simulink model "component_model"  (R2019a)
settings: Solver=VariableStepAuto  StartTime=0.0  StopTime=10.0  RelTol=1e-3
settings Model: Creator=anton  LastModifiedBy=anton

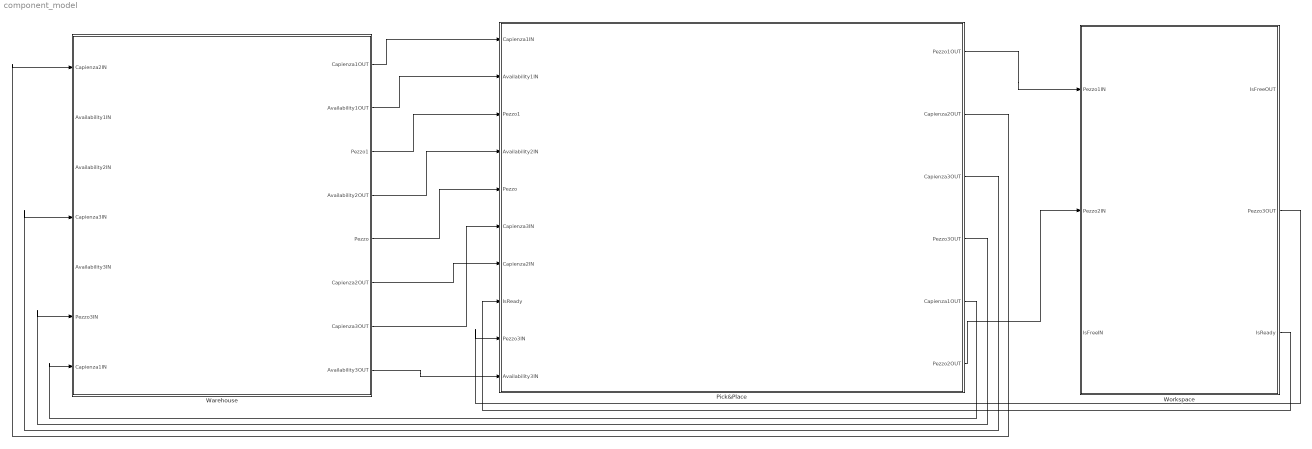
== system component_model ==
  Pick&Place : Subsystem
      settings: PortSchema="{\"entries\":[{\"content\":{\"headerSize\":26,\"margin\":15,\"minimumSpacing\":25,\"sides\":[{\"content\":{\"connectorIds\":[\"In1\",\"In2\",\"In3\",\"In4\",\"In5\",\"In6\",\"In7\",\"In8\",\"In9\",\"In10\"]},\"type\":\"ConnectorPlacement.EquallySpacedRectSide\",\"uuid\":\"cd5611c0-8a30-4803-bae5-8792d5ed3138\"},{\"content\":{\"connectorIds\":[\"Out1\",\"Out2\",\"Out3\",\"Out4\",\"Out5\",\"Out6\"],\"side\":\"RIGHT\"},\"type\":\"ConnectorPlacement.EquallySpacedRectSide\",\"uuid\":\"19615e04-708c-4dc8-9217-130af3d4c815\"},{\"content\":{\"connectorIds\":[],\"side\":\"TOP\"},\"type\":\"ConnectorPlacement.EquallySpacedRectSide\",\"uuid\":\"bde4fae3-4c2b-4ff8-8efa-5dc73cdd4226\"}]},\"type\":\"ConnectorPlacement.EquallySpacedConnector\",\"uuid\":\"74f0ebde-c382-4fb1-af99-ecf6372bc12c\"}],\"packageUris\":[\"http:\\/\\/schema.mathworks.com\\/mf0\\/Connector\\/19700101\"],\"version\":\"1.0\"}"
  Warehouse : Subsystem
      settings: PortSchema="{\"entries\":[{\"content\":{\"headerSize\":26,\"margin\":15,\"minimumSpacing\":25,\"sides\":[{\"content\":{\"connectorIds\":[\"In1\",\"In2\",\"In3\",\"In4\",\"In5\",\"In6\",\"In7\"]},\"type\":\"ConnectorPlacement.EquallySpacedRectSide\",\"uuid\":\"cd5611c0-8a30-4803-bae5-8792d5ed3138\"},{\"content\":{\"connectorIds\":[\"Out1\",\"Out2\",\"Out3\",\"Out4\",\"Out5\",\"Out6\",\"Out7\",\"Out8\"],\"side\":\"RIGHT\"},\"type\":\"ConnectorPlacement.EquallySpacedRectSide\",\"uuid\":\"19615e04-708c-4dc8-9217-130af3d4c815\"},{\"content\":{\"connectorIds\":[],\"side\":\"TOP\"},\"type\":\"ConnectorPlacement.EquallySpacedRectSide\",\"uuid\":\"bde4fae3-4c2b-4ff8-8efa-5dc73cdd4226\"}]},\"type\":\"ConnectorPlacement.EquallySpacedConnector\",\"uuid\":\"74f0ebde-c382-4fb1-af99-ecf6372bc12c\"}],\"packageUris\":[\"http:\\/\\/schema.mathworks.com\\/mf0\\/Connector\\/19700101\"],\"version\":\"1.0\"}"
  Workspace : Subsystem
      settings: PortSchema="{\"entries\":[{\"content\":{\"headerSize\":26,\"margin\":15,\"minimumSpacing\":25,\"sides\":[{\"content\":{\"connectorIds\":[\"In1\",\"In2\",\"In3\"]},\"type\":\"ConnectorPlacement.EquallySpacedRectSide\",\"uuid\":\"cd5611c0-8a30-4803-bae5-8792d5ed3138\"},{\"content\":{\"connectorIds\":[\"Out1\",\"Out2\",\"Out3\"],\"side\":\"RIGHT\"},\"type\":\"ConnectorPlacement.EquallySpacedRectSide\",\"uuid\":\"19615e04-708c-4dc8-9217-130af3d4c815\"},{\"content\":{\"connectorIds\":[],\"side\":\"TOP\"},\"type\":\"ConnectorPlacement.EquallySpacedRectSide\",\"uuid\":\"bde4fae3-4c2b-4ff8-8efa-5dc73cdd4226\"}]},\"type\":\"ConnectorPlacement.EquallySpacedConnector\",\"uuid\":\"74f0ebde-c382-4fb1-af99-ecf6372bc12c\"}],\"packageUris\":[\"http:\\/\\/schema.mathworks.com\\/mf0\\/Connector\\/19700101\"],\"version\":\"1.0\"}"
  wires:
  Pick&Place/5(Capienza1OUT) -> Warehouse/7(Capienza1IN)
  Pick&Place/2(Capienza2OUT) -> Warehouse/1(Capienza2IN)
  Pick&Place/3(Capienza3OUT) -> Warehouse/4(Capienza3IN)
  Warehouse/1(Capienza1OUT) -> Pick&Place/1(Capienza1IN)
  Warehouse/6(Capienza2OUT) -> Pick&Place/7(Capienza2IN)
  Warehouse/3(Pezzo1) -> Pick&Place/3(Pezzo1)
  Warehouse/5(Pezzo) -> Pick&Place/5(Pezzo)
  Warehouse/2(Availability1OUT) -> Pick&Place/2(Availability1IN)
  Warehouse/4(Availability2OUT) -> Pick&Place/4(Availability2IN)
  Warehouse/7(Capienza3OUT) -> Pick&Place/6(Capienza3IN)
  Pick&Place/1(Pezzo1OUT) -> Workspace/1(Pezzo1IN)
  Pick&Place/6(Pezzo2OUT) -> Workspace/2(Pezzo2IN)
  Workspace/3(IsReady) -> Pick&Place/8(IsReady)
  Workspace/2(Pezzo3OUT) -> Pick&Place/9(Pezzo3IN)
  Pick&Place/4(Pezzo3OUT) -> Warehouse/6(Pezzo3IN)
  Warehouse/8(Availability3OUT) -> Pick&Place/10(Availability3IN)

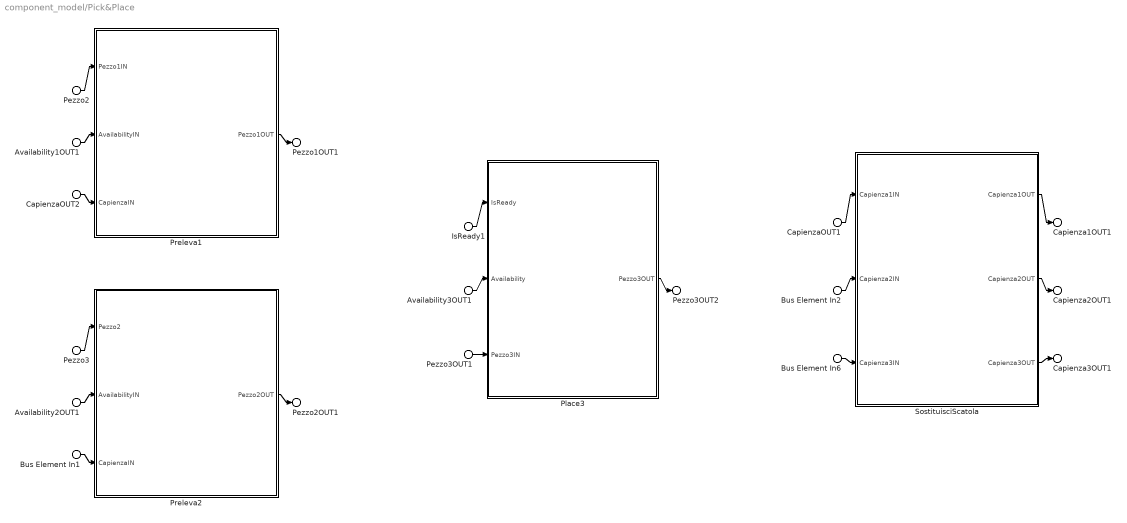
== system component_model/Pick&Place ==
  CapienzaOUT1 : Inport  PortName=Capienza1IN
  CapienzaOUT2 : Inport  PortName=Capienza1IN
  Availability1OUT1 : Inport  Port=2  PortName=Availability1IN
  Pezzo2 : Inport  Port=3  PortName=Pezzo1
  Availability2OUT1 : Inport  Port=4  PortName=Availability2IN
  Pezzo3 : Inport  Port=5  PortName=Pezzo
  Bus Element In6 : Inport  Port=6  PortName=Capienza3IN
  Bus Element In2 : Inport  Port=7  PortName=Capienza2IN
  Bus Element In1 : Inport  Port=7  PortName=Capienza2IN
  IsReady1 : Inport  Port=8  PortName=IsReady
  Pezzo3OUT1 : Inport  Port=9  PortName=Pezzo3IN
  Availability3OUT1 : Inport  Port=10  PortName=Availability3IN
  Place3 : Subsystem
      settings: PortSchema="{\"entries\":[{\"content\":{\"headerSize\":26,\"margin\":15,\"minimumSpacing\":25,\"sides\":[{\"content\":{\"connectorIds\":[\"In1\",\"In2\",\"In3\"]},\"type\":\"ConnectorPlacement.EquallySpacedRectSide\",\"uuid\":\"cd5611c0-8a30-4803-bae5-8792d5ed3138\"},{\"content\":{\"connectorIds\":[\"Out1\"],\"side\":\"RIGHT\"},\"type\":\"ConnectorPlacement.EquallySpacedRectSide\",\"uuid\":\"19615e04-708c-4dc8-9217-130af3d4c815\"},{\"content\":{\"connectorIds\":[],\"side\":\"TOP\"},\"type\":\"ConnectorPlacement.EquallySpacedRectSide\",\"uuid\":\"bde4fae3-4c2b-4ff8-8efa-5dc73cdd4226\"},{\"content\":{\"connectorIds\":[],\"side\":\"BOTTOM\"},\"type\":\"ConnectorPlacement.EquallySpacedRectSide\",\"uuid\":\"1c0666f0-126c-43a7-b404-605aac664503\"}]},\"type\":\"ConnectorPlacement.EquallySpacedConnector\",\"uuid\":\"74f0ebde-c382-4fb1-af99-ecf6372bc12c\"}],\"packageUris\":[\"http:\\/\\/schema.mathworks.com\\/mf0\\/Connector\\/19700101\"],\"version\":\"1.0\"}"
  Preleva1 : Subsystem
      settings: PortSchema="{\"entries\":[{\"content\":{\"headerSize\":26,\"margin\":15,\"minimumSpacing\":25,\"sides\":[{\"content\":{\"connectorIds\":[\"In1\",\"In2\",\"In3\"]},\"type\":\"ConnectorPlacement.EquallySpacedRectSide\",\"uuid\":\"cd5611c0-8a30-4803-bae5-8792d5ed3138\"},{\"content\":{\"connectorIds\":[\"Out1\"],\"side\":\"RIGHT\"},\"type\":\"ConnectorPlacement.EquallySpacedRectSide\",\"uuid\":\"19615e04-708c-4dc8-9217-130af3d4c815\"},{\"content\":{\"connectorIds\":[],\"side\":\"TOP\"},\"type\":\"ConnectorPlacement.EquallySpacedRectSide\",\"uuid\":\"bde4fae3-4c2b-4ff8-8efa-5dc73cdd4226\"}]},\"type\":\"ConnectorPlacement.EquallySpacedConnector\",\"uuid\":\"74f0ebde-c382-4fb1-af99-ecf6372bc12c\"}],\"packageUris\":[\"http:\\/\\/schema.mathworks.com\\/mf0\\/Connector\\/19700101\"],\"version\":\"1.0\"}"
  Preleva2 : Subsystem
      settings: PortSchema="{\"entries\":[{\"content\":{\"headerSize\":26,\"margin\":15,\"minimumSpacing\":25,\"sides\":[{\"content\":{\"connectorIds\":[\"In1\",\"In2\",\"In3\"]},\"type\":\"ConnectorPlacement.EquallySpacedRectSide\",\"uuid\":\"cd5611c0-8a30-4803-bae5-8792d5ed3138\"},{\"content\":{\"connectorIds\":[\"Out1\"],\"side\":\"RIGHT\"},\"type\":\"ConnectorPlacement.EquallySpacedRectSide\",\"uuid\":\"19615e04-708c-4dc8-9217-130af3d4c815\"},{\"content\":{\"connectorIds\":[],\"side\":\"TOP\"},\"type\":\"ConnectorPlacement.EquallySpacedRectSide\",\"uuid\":\"bde4fae3-4c2b-4ff8-8efa-5dc73cdd4226\"}]},\"type\":\"ConnectorPlacement.EquallySpacedConnector\",\"uuid\":\"74f0ebde-c382-4fb1-af99-ecf6372bc12c\"}],\"packageUris\":[\"http:\\/\\/schema.mathworks.com\\/mf0\\/Connector\\/19700101\"],\"version\":\"1.0\"}"
  SostituisciScatola : Subsystem
      settings: PortSchema="{\"entries\":[{\"content\":{\"headerSize\":26,\"margin\":15,\"minimumSpacing\":25,\"sides\":[{\"content\":{\"connectorIds\":[\"In1\",\"In2\",\"In3\"]},\"type\":\"ConnectorPlacement.EquallySpacedRectSide\",\"uuid\":\"cd5611c0-8a30-4803-bae5-8792d5ed3138\"},{\"content\":{\"connectorIds\":[\"Out1\",\"Out2\",\"Out3\"],\"side\":\"RIGHT\"},\"type\":\"ConnectorPlacement.EquallySpacedRectSide\",\"uuid\":\"19615e04-708c-4dc8-9217-130af3d4c815\"},{\"content\":{\"connectorIds\":[],\"side\":\"TOP\"},\"type\":\"ConnectorPlacement.EquallySpacedRectSide\",\"uuid\":\"bde4fae3-4c2b-4ff8-8efa-5dc73cdd4226\"}]},\"type\":\"ConnectorPlacement.EquallySpacedConnector\",\"uuid\":\"74f0ebde-c382-4fb1-af99-ecf6372bc12c\"}],\"packageUris\":[\"http:\\/\\/schema.mathworks.com\\/mf0\\/Connector\\/19700101\"],\"version\":\"1.0\"}"
  Pezzo1OUT1 : Outport  PortName=Pezzo1OUT
  Capienza2OUT1 : Outport  Port=2  PortName=Capienza2OUT
  Capienza3OUT1 : Outport  Port=3  PortName=Capienza3OUT
  Pezzo3OUT2 : Outport  Port=4  PortName=Pezzo3OUT
  Capienza1OUT1 : Outport  Port=5  PortName=Capienza1OUT
  Pezzo2OUT1 : Outport  Port=6  PortName=Pezzo2OUT
  wires:
  SostituisciScatola/1(Capienza1OUT) -> Capienza1OUT1/1
  SostituisciScatola/2(Capienza2OUT) -> Capienza2OUT1/1
  SostituisciScatola/3(Capienza3OUT) -> Capienza3OUT1/1
  CapienzaOUT1/1 -> SostituisciScatola/1(Capienza1IN)
  Bus Element In2/1 -> SostituisciScatola/2(Capienza2IN)
  CapienzaOUT2/1 -> Preleva1/3(CapienzaIN)
  Bus Element In1/1 -> Preleva2/3(CapienzaIN)
  Pezzo2/1 -> Preleva1/1(Pezzo1IN)
  Pezzo3/1 -> Preleva2/1(Pezzo2)
  Availability1OUT1/1 -> Preleva1/2(AvailabilityIN)
  Availability2OUT1/1 -> Preleva2/2(AvailabilityIN)
  Preleva1/1(Pezzo1OUT) -> Pezzo1OUT1/1
  Preleva2/1(Pezzo2OUT) -> Pezzo2OUT1/1
  Bus Element In6/1 -> SostituisciScatola/3(Capienza3IN)
  IsReady1/1 -> Place3/1(IsReady)
  Pezzo3OUT1/1 -> Place3/3(Pezzo3IN)
  Place3/1(Pezzo3OUT) -> Pezzo3OUT2/1
  Availability3OUT1/1 -> Place3/2(Availability)

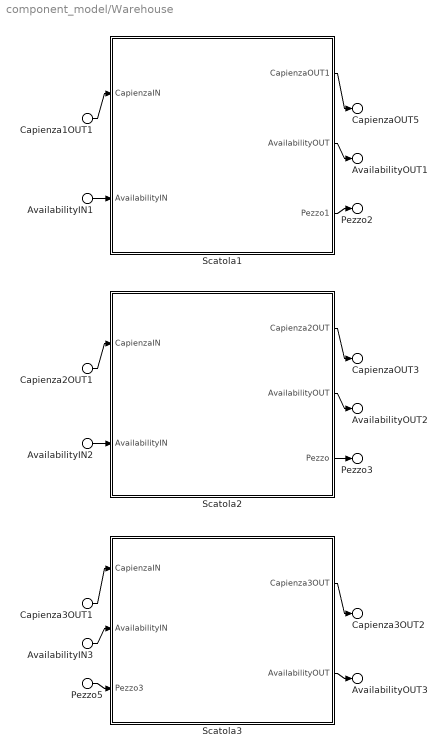
== system component_model/Warehouse ==
  Capienza2OUT1 : Inport  PortName=Capienza2IN
  AvailabilityIN1 : Inport  Port=2  PortName=Availability1IN
  AvailabilityIN2 : Inport  Port=3  PortName=Availability2IN
  Capienza3OUT1 : Inport  Port=4  PortName=Capienza3IN
  AvailabilityIN3 : Inport  Port=5  PortName=Availability3IN
  Pezzo5 : Inport  Port=6  PortName=Pezzo3IN
  Capienza1OUT1 : Inport  Port=7  PortName=Capienza1IN
  Scatola1 : Subsystem
      settings: PortSchema="{\"entries\":[{\"content\":{\"headerSize\":26,\"margin\":15,\"minimumSpacing\":25,\"sides\":[{\"content\":{\"connectorIds\":[\"In1\",\"In2\"]},\"type\":\"ConnectorPlacement.EquallySpacedRectSide\",\"uuid\":\"cd5611c0-8a30-4803-bae5-8792d5ed3138\"},{\"content\":{\"connectorIds\":[\"Out1\",\"Out2\",\"Out3\"],\"side\":\"RIGHT\"},\"type\":\"ConnectorPlacement.EquallySpacedRectSide\",\"uuid\":\"19615e04-708c-4dc8-9217-130af3d4c815\"},{\"content\":{\"connectorIds\":[],\"side\":\"TOP\"},\"type\":\"ConnectorPlacement.EquallySpacedRectSide\",\"uuid\":\"bde4fae3-4c2b-4ff8-8efa-5dc73cdd4226\"}]},\"type\":\"ConnectorPlacement.EquallySpacedConnector\",\"uuid\":\"74f0ebde-c382-4fb1-af99-ecf6372bc12c\"}],\"packageUris\":[\"http:\\/\\/schema.mathworks.com\\/mf0\\/Connector\\/19700101\"],\"version\":\"1.0\"}"
  Scatola2 : Subsystem
      settings: PortSchema="{\"entries\":[{\"content\":{\"headerSize\":26,\"margin\":15,\"minimumSpacing\":25,\"sides\":[{\"content\":{\"connectorIds\":[\"In1\",\"In2\"]},\"type\":\"ConnectorPlacement.EquallySpacedRectSide\",\"uuid\":\"cd5611c0-8a30-4803-bae5-8792d5ed3138\"},{\"content\":{\"connectorIds\":[\"Out1\",\"Out2\",\"Out3\"],\"side\":\"RIGHT\"},\"type\":\"ConnectorPlacement.EquallySpacedRectSide\",\"uuid\":\"19615e04-708c-4dc8-9217-130af3d4c815\"},{\"content\":{\"connectorIds\":[],\"side\":\"TOP\"},\"type\":\"ConnectorPlacement.EquallySpacedRectSide\",\"uuid\":\"bde4fae3-4c2b-4ff8-8efa-5dc73cdd4226\"}]},\"type\":\"ConnectorPlacement.EquallySpacedConnector\",\"uuid\":\"74f0ebde-c382-4fb1-af99-ecf6372bc12c\"}],\"packageUris\":[\"http:\\/\\/schema.mathworks.com\\/mf0\\/Connector\\/19700101\"],\"version\":\"1.0\"}"
  Scatola3 : Subsystem
      settings: PortSchema="{\"entries\":[{\"content\":{\"headerSize\":26,\"margin\":15,\"minimumSpacing\":25,\"sides\":[{\"content\":{\"connectorIds\":[\"In1\",\"In2\",\"In3\"]},\"type\":\"ConnectorPlacement.EquallySpacedRectSide\",\"uuid\":\"cd5611c0-8a30-4803-bae5-8792d5ed3138\"},{\"content\":{\"connectorIds\":[\"Out1\",\"Out2\"],\"side\":\"RIGHT\"},\"type\":\"ConnectorPlacement.EquallySpacedRectSide\",\"uuid\":\"19615e04-708c-4dc8-9217-130af3d4c815\"},{\"content\":{\"connectorIds\":[],\"side\":\"TOP\"},\"type\":\"ConnectorPlacement.EquallySpacedRectSide\",\"uuid\":\"bde4fae3-4c2b-4ff8-8efa-5dc73cdd4226\"}]},\"type\":\"ConnectorPlacement.EquallySpacedConnector\",\"uuid\":\"74f0ebde-c382-4fb1-af99-ecf6372bc12c\"}],\"packageUris\":[\"http:\\/\\/schema.mathworks.com\\/mf0\\/Connector\\/19700101\"],\"version\":\"1.0\"}"
  CapienzaOUT5 : Outport  PortName=Capienza1OUT
  AvailabilityOUT1 : Outport  Port=2  PortName=Availability1OUT
  Pezzo2 : Outport  Port=3  PortName=Pezzo1
  AvailabilityOUT2 : Outport  Port=4  PortName=Availability2OUT
  Pezzo3 : Outport  Port=5  PortName=Pezzo
  CapienzaOUT3 : Outport  Port=6  PortName=Capienza2OUT
  Capienza3OUT2 : Outport  Port=7  PortName=Capienza3OUT
  AvailabilityOUT3 : Outport  Port=8  PortName=Availability3OUT
  wires:
  Capienza3OUT1/1 -> Scatola3/1(CapienzaIN)
  Capienza1OUT1/1 -> Scatola1/1(CapienzaIN)
  Capienza2OUT1/1 -> Scatola2/1(CapienzaIN)
  Scatola2/1(Capienza2OUT) -> CapienzaOUT3/1
  Scatola1/1(CapienzaOUT1) -> CapienzaOUT5/1
  Scatola1/2(AvailabilityOUT) -> AvailabilityOUT1/1
  Scatola2/2(AvailabilityOUT) -> AvailabilityOUT2/1
  Scatola3/2(AvailabilityOUT) -> AvailabilityOUT3/1
  Scatola1/3(Pezzo1) -> Pezzo2/1
  Scatola2/3(Pezzo) -> Pezzo3/1
  Scatola3/1(Capienza3OUT) -> Capienza3OUT2/1
  AvailabilityIN1/1 -> Scatola1/2(AvailabilityIN)
  AvailabilityIN2/1 -> Scatola2/2(AvailabilityIN)
  AvailabilityIN3/1 -> Scatola3/2(AvailabilityIN)
  Pezzo5/1 -> Scatola3/3(Pezzo3)

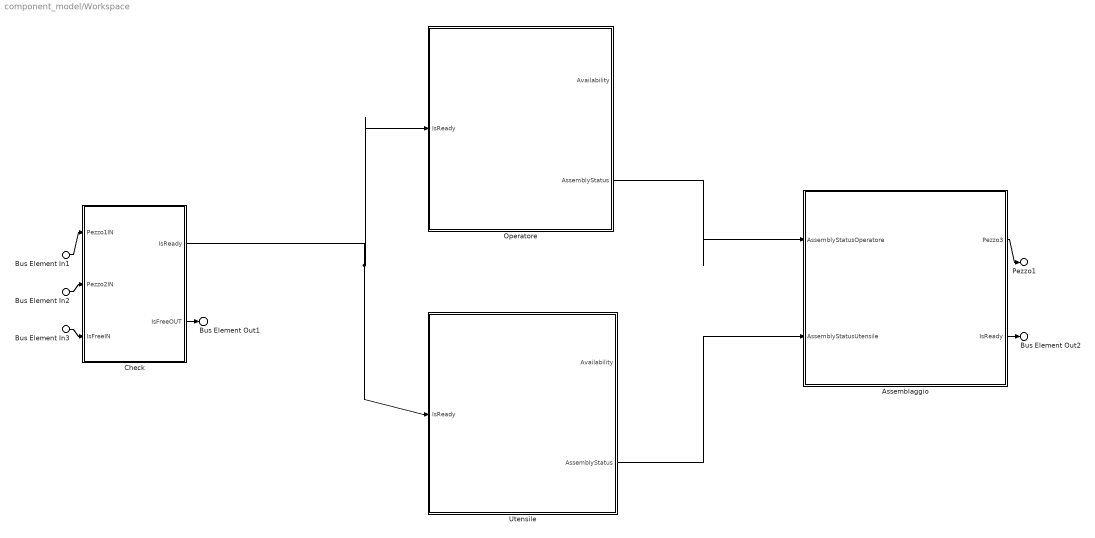
== system component_model/Workspace ==
  Bus Element In1 : Inport  PortName=Pezzo1IN
  Bus Element In2 : Inport  Port=2  PortName=Pezzo2IN
  Bus Element In3 : Inport  Port=3  PortName=IsFreeIN
  Assemblaggio : Subsystem
      settings: PortSchema="{\"entries\":[{\"content\":{\"headerSize\":26,\"margin\":15,\"minimumSpacing\":25,\"sides\":[{\"content\":{\"connectorIds\":[\"In1\",\"In2\"]},\"type\":\"ConnectorPlacement.EquallySpacedRectSide\",\"uuid\":\"cd5611c0-8a30-4803-bae5-8792d5ed3138\"},{\"content\":{\"connectorIds\":[\"Out1\",\"Out2\"],\"side\":\"RIGHT\"},\"type\":\"ConnectorPlacement.EquallySpacedRectSide\",\"uuid\":\"19615e04-708c-4dc8-9217-130af3d4c815\"},{\"content\":{\"connectorIds\":[],\"side\":\"TOP\"},\"type\":\"ConnectorPlacement.EquallySpacedRectSide\",\"uuid\":\"bde4fae3-4c2b-4ff8-8efa-5dc73cdd4226\"}]},\"type\":\"ConnectorPlacement.EquallySpacedConnector\",\"uuid\":\"74f0ebde-c382-4fb1-af99-ecf6372bc12c\"}],\"packageUris\":[\"http:\\/\\/schema.mathworks.com\\/mf0\\/Connector\\/19700101\"],\"version\":\"1.0\"}"
  Check : Subsystem
      settings: PortSchema="{\"entries\":[{\"content\":{\"headerSize\":26,\"margin\":15,\"minimumSpacing\":25,\"sides\":[{\"content\":{\"connectorIds\":[\"In1\",\"In2\",\"In3\"]},\"type\":\"ConnectorPlacement.EquallySpacedRectSide\",\"uuid\":\"cd5611c0-8a30-4803-bae5-8792d5ed3138\"},{\"content\":{\"connectorIds\":[\"Out1\",\"Out2\"],\"side\":\"RIGHT\"},\"type\":\"ConnectorPlacement.EquallySpacedRectSide\",\"uuid\":\"19615e04-708c-4dc8-9217-130af3d4c815\"},{\"content\":{\"connectorIds\":[],\"side\":\"TOP\"},\"type\":\"ConnectorPlacement.EquallySpacedRectSide\",\"uuid\":\"bde4fae3-4c2b-4ff8-8efa-5dc73cdd4226\"}]},\"type\":\"ConnectorPlacement.EquallySpacedConnector\",\"uuid\":\"74f0ebde-c382-4fb1-af99-ecf6372bc12c\"}],\"packageUris\":[\"http:\\/\\/schema.mathworks.com\\/mf0\\/Connector\\/19700101\"],\"version\":\"1.0\"}"
  Operatore : Subsystem
      settings: PortSchema="{\"entries\":[{\"content\":{\"headerSize\":26,\"margin\":15,\"minimumSpacing\":25,\"sides\":[{\"content\":{\"connectorIds\":[\"In1\"]},\"type\":\"ConnectorPlacement.EquallySpacedRectSide\",\"uuid\":\"cd5611c0-8a30-4803-bae5-8792d5ed3138\"},{\"content\":{\"connectorIds\":[\"Out1\",\"Out2\"],\"side\":\"RIGHT\"},\"type\":\"ConnectorPlacement.EquallySpacedRectSide\",\"uuid\":\"19615e04-708c-4dc8-9217-130af3d4c815\"},{\"content\":{\"connectorIds\":[],\"side\":\"TOP\"},\"type\":\"ConnectorPlacement.EquallySpacedRectSide\",\"uuid\":\"bde4fae3-4c2b-4ff8-8efa-5dc73cdd4226\"}]},\"type\":\"ConnectorPlacement.EquallySpacedConnector\",\"uuid\":\"74f0ebde-c382-4fb1-af99-ecf6372bc12c\"}],\"packageUris\":[\"http:\\/\\/schema.mathworks.com\\/mf0\\/Connector\\/19700101\"],\"version\":\"1.0\"}"
  Utensile : Subsystem
      settings: PortSchema="{\"entries\":[{\"content\":{\"headerSize\":26,\"margin\":15,\"minimumSpacing\":25,\"sides\":[{\"content\":{\"connectorIds\":[\"In1\"]},\"type\":\"ConnectorPlacement.EquallySpacedRectSide\",\"uuid\":\"cd5611c0-8a30-4803-bae5-8792d5ed3138\"},{\"content\":{\"connectorIds\":[\"Out1\",\"Out2\"],\"side\":\"RIGHT\"},\"type\":\"ConnectorPlacement.EquallySpacedRectSide\",\"uuid\":\"19615e04-708c-4dc8-9217-130af3d4c815\"},{\"content\":{\"connectorIds\":[],\"side\":\"TOP\"},\"type\":\"ConnectorPlacement.EquallySpacedRectSide\",\"uuid\":\"bde4fae3-4c2b-4ff8-8efa-5dc73cdd4226\"}]},\"type\":\"ConnectorPlacement.EquallySpacedConnector\",\"uuid\":\"74f0ebde-c382-4fb1-af99-ecf6372bc12c\"}],\"packageUris\":[\"http:\\/\\/schema.mathworks.com\\/mf0\\/Connector\\/19700101\"],\"version\":\"1.0\"}"
  Bus Element Out1 : Outport  PortName=IsFreeOUT
  Pezzo1 : Outport  Port=2  PortName=Pezzo3OUT
  Bus Element Out2 : Outport  Port=3  PortName=IsReady
  wires:
  Operatore/2(AssemblyStatus) -> Assemblaggio/1(AssemblyStatusOperatore)
  Utensile/2(AssemblyStatus) -> Assemblaggio/2(AssemblyStatusUtensile)
  Bus Element In1/1 -> Check/1(Pezzo1IN)
  Bus Element In2/1 -> Check/2(Pezzo2IN)
  Check/1(IsReady) -> Utensile/1(IsReady), Operatore/1(IsReady)
  Assemblaggio/1(Pezzo3) -> Pezzo1/1
  Assemblaggio/2(IsReady) -> Bus Element Out2/1
  Bus Element In3/1 -> Check/3(IsFreeIN)
  Check/2(IsFreeOUT) -> Bus Element Out1/1

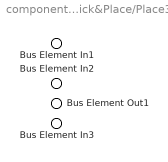
== system component_model/Pick&Place/Place3 ==
  Bus Element In1 : Inport  PortName=IsReady
  Bus Element In2 : Inport  Port=2  PortName=Availability
  Bus Element In3 : Inport  Port=3  PortName=Pezzo3IN
  Bus Element Out1 : Outport  PortName=Pezzo3OUT

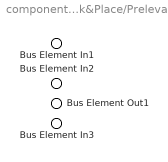
== system component_model/Pick&Place/Preleva1 ==
  Bus Element In1 : Inport  PortName=Pezzo1IN
  Bus Element In2 : Inport  Port=2  PortName=AvailabilityIN
  Bus Element In3 : Inport  Port=3  PortName=CapienzaIN
  Bus Element Out1 : Outport  PortName=Pezzo1OUT

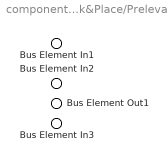
== system component_model/Pick&Place/Preleva2 ==
  Bus Element In1 : Inport  PortName=Pezzo2
  Bus Element In2 : Inport  Port=2  PortName=AvailabilityIN
  Bus Element In3 : Inport  Port=3  PortName=CapienzaIN
  Bus Element Out1 : Outport  PortName=Pezzo2OUT

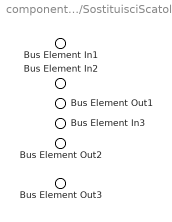
== system component_model/Pick&Place/SostituisciScatola ==
  Bus Element In1 : Inport  PortName=Capienza1IN
  Bus Element In2 : Inport  Port=2  PortName=Capienza2IN
  Bus Element In3 : Inport  Port=3  PortName=Capienza3IN
  Bus Element Out1 : Outport  PortName=Capienza1OUT
  Bus Element Out2 : Outport  Port=2  PortName=Capienza2OUT
  Bus Element Out3 : Outport  Port=3  PortName=Capienza3OUT

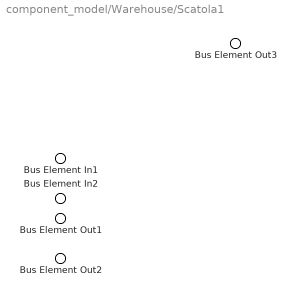
== system component_model/Warehouse/Scatola1 ==
  Bus Element In1 : Inport  PortName=CapienzaIN
  Bus Element In2 : Inport  Port=2  PortName=AvailabilityIN
  Bus Element Out1 : Outport  PortName=CapienzaOUT1
  Bus Element Out3 : Outport  Port=2  PortName=AvailabilityOUT
  Bus Element Out2 : Outport  Port=3  PortName=Pezzo1

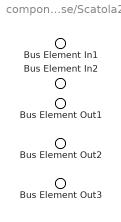
== system component_model/Warehouse/Scatola2 ==
  Bus Element In1 : Inport  PortName=CapienzaIN
  Bus Element In2 : Inport  Port=2  PortName=AvailabilityIN
  Bus Element Out1 : Outport  PortName=Capienza2OUT
  Bus Element Out2 : Outport  Port=2  PortName=AvailabilityOUT
  Bus Element Out3 : Outport  Port=3  PortName=Pezzo

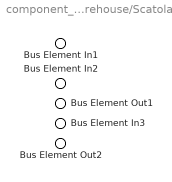
== system component_model/Warehouse/Scatola3 ==
  Bus Element In1 : Inport  PortName=CapienzaIN
  Bus Element In2 : Inport  Port=2  PortName=AvailabilityIN
  Bus Element In3 : Inport  Port=3  PortName=Pezzo3
  Bus Element Out1 : Outport  PortName=Capienza3OUT
  Bus Element Out2 : Outport  Port=2  PortName=AvailabilityOUT

== system component_model/Workspace/Assemblaggio ==
  Bus Element In1 : Inport  PortName=AssemblyStatusOperatore
  Bus Element In2 : Inport  Port=2  PortName=AssemblyStatusUtensile
  Bus Element Out1 : Outport  PortName=Pezzo3
  Bus Element Out2 : Outport  Port=2  PortName=IsReady

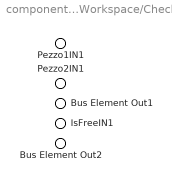
== system component_model/Workspace/Check ==
  Pezzo1IN1 : Inport  PortName=Pezzo1IN
  Pezzo2IN1 : Inport  Port=2  PortName=Pezzo2IN
  IsFreeIN1 : Inport  Port=3  PortName=IsFreeIN
  Bus Element Out1 : Outport  PortName=IsReady
  Bus Element Out2 : Outport  Port=2  PortName=IsFreeOUT

== system component_model/Workspace/Operatore ==
  Bus Element In1 : Inport  PortName=IsReady
  Bus Element Out1 : Outport  PortName=Availability
  Bus Element Out2 : Outport  Port=2  PortName=AssemblyStatus

== system component_model/Workspace/Utensile ==
  Bus Element In1 : Inport  PortName=IsReady
  Bus Element Out1 : Outport  PortName=Availability
  Bus Element Out2 : Outport  Port=2  PortName=AssemblyStatus
